simulink library "mbed_targets_stm_disco_f746"  (R2015a)
settings: Solver=ode45  StartTime=0.0  StopTime=10.0  RelTol=1e-3
libraries: mbed_targets_stm_disco_f407 x9, mbed_lib x3
settings Model: CovSFcnEnable=off  Creator=oh  LastModifiedBy=Stuv
settings DebuggingCC: SolverPrmCheckMsg=warning

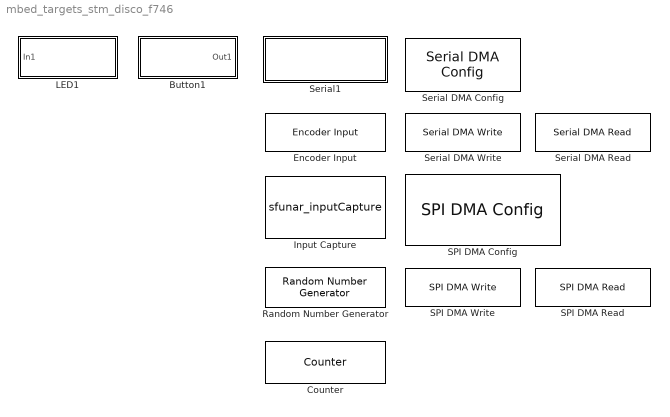
== system mbed_targets_stm_disco_f746 ==
  Button1 : Subsystem  mask{Parameter1=0}
      mask Display:
      | plot([0 0.15 0.15 0.35 0.35 0.5],[0.3 0.3 0.7 0.7 0.3 0.3])
      | port_label('output',1,['UsrBtn1']);
  Counter : mbed_targets_stm_disco_f407/Counter  TimerNumber=1  InputChannel=TI1 rising  TiPort=A  TiPin=0  TiPupd=PullNone  MaxCnt=10  Interrupt=no interrupt generation  RstEnable=off
  Encoder Input : mbed_targets_stm_disco_f407/Encoder Input  TimerNumber=TIM1  EncoderMode=TI1  Ti1Port=A  Ti1Pin=0  Ti2Port=A  Ti2Pin=0  InputMode=PullNone  Resolution=65535  SampleTime=-1
  Input Capture : S-Function  FunctionName=sfunar_inputCapture  Parameters=SampleTime, TimerNumber, Frequency, Ti1Active, Ti1Port, Ti1Pin, Ti1Pupd, Ti2Active, Ti2Port, Ti2Pin, Ti2Pupd, Ti3Active, Ti3Port, Ti3Pin, Ti3Pupd, Ti4Active, Ti4Port, Ti4Pin, Ti4Pupd, OutputMode  mask{TimerNumber=1, Frequency=1000000, OutputMode=Raw, Ti1Active=Rising, Ti1Port=A, Ti1Pin=0, Ti1Pupd=PullNone, Ti2Active=None, Ti2Port=A, Ti2Pin=0, Ti2Pupd=PullNone, Ti3Active=None, Ti3Port=A, Ti3Pin=0, Ti3Pupd=PullNone, Ti4Active=None, Ti4Port=A, Ti4Pin=0, Ti4Pupd=PullNone, SampleTime=-1}
      mask prompts: TimerNumber "Timer"; OutputMode "Output mode"; Ti1Active "Activate TI1"; Ti1Port "TI1 Port"; Ti1Pin "TI1 Pin"; Ti1Pupd "TI1 Pull type"; Ti2Active "Activate TI2"; Ti2Port "TI2 Port"; Ti2Pin "TI2 Pin"; Ti2Pupd "Ti2 Pull type"; Ti3Active "Activate TI3"; Ti3Port "TI3 Port"; Ti3Pin "TI3 Pin"; Ti3Pupd "TI3 Pull type"; Ti4Active "Activate TI4"; Ti4Port "TI4 Port"; Ti4Pin "TI4 Pin"; Ti4Pupd "TI4 Pull type"; SampleTime "Sample time (-1 for inherited):"
      mask TypeOptions TimerNumber: 1 | 2 | 3 | 4 | 5 | 8 | 9 | 10 | 11 | 12 | 13 | 14 | 15 | 16 | 17 | 20
      mask TypeOptions OutputMode: Raw | Period | Frequency | High Pulse | Low Pulse
      mask TypeOptions Ti1Active: None | Rising | Falling | Both
      mask TypeOptions Ti1Port: A | B | C | D | E | F
      mask TypeOptions Ti1Pin: 0 | 1 | 2 | 3 | 4 | 5 | 6 | 7 | 8 | 9 | 10 | 11 | 12 | 13 | 14 | 15
      mask TypeOptions Ti1Pupd: PullNone | PullUp | PullDown
      mask TypeOptions Ti2Active: None | Rising | Falling | Both
      mask TypeOptions Ti2Port: A | B | C | D | E | F
      mask TypeOptions Ti2Pin: 0 | 1 | 2 | 3 | 4 | 5 | 6 | 7 | 8 | 9 | 10 | 11 | 12 | 13 | 14 | 15
      mask TypeOptions Ti2Pupd: PullNone | PullUp | PullDown
      mask TypeOptions Ti3Active: None | Rising | Falling | Both
      mask TypeOptions Ti3Port: A | B | C | D | E | F
      mask TypeOptions Ti3Pin: 0 | 1 | 2 | 3 | 4 | 5 | 6 | 7 | 8 | 9 | 10 | 11 | 12 | 13 | 14 | 15
      mask TypeOptions Ti3Pupd: PullNone | PullUp | PullDown
      mask TypeOptions Ti4Active: None | Rising | Falling | Both
      mask TypeOptions Ti4Port: A | B | C | D | E | F
      mask TypeOptions Ti4Pin: 0 | 1 | 2 | 3 | 4 | 5 | 6 | 7 | 8 | 9 | 10 | 11 | 12 | 13 | 14 | 15
      mask TypeOptions Ti4Pupd: PullNone | PullUp | PullDown
      mask Display:
      | disp(['Timer ' num2str(TimerNumber) '\n']);
      | disp('\n Input Capture');
      | port = 1;
      | 
      | if Ti1Active > 1
      |     port_label('output',port,['P' Ti1Port+64 '.' num2str(Ti1Pin-1)]);
      |     port = port + 1;
      | end
      | 
      | if Ti2Active > 1
      |     port_label('output',port,['P' Ti2Port+64 '.' num2str(Ti2Pin-1)]);
      |     port = port + 1;
      | end
      | 
      | if Ti3Active > 1
      |     port_label('output',port,['P' Ti3Port+64 '.' num2str(Ti3Pin-1)]);
      |     port = port + 1;
      | end
      | 
      | if Ti4Active > 1
      |     port_label('output',port,['P' Ti4Port+64 '.' num2str(Ti4Pin-1)]);
      |     port = port + 1;
      | end
  LED1 : Subsystem  mask{Parameter1=0}
      mask Display:
      | plot([0.5 0.65 0.65 0.85 0.85 1],[0.3 0.3 0.7 0.7 0.3 0.3])
      | port_label('input',1,['LED1']);
  Random Number Generator : mbed_targets_stm_disco_f407/Random Number Generator  SampleTime=-1
  SPI DMA Config : mbed_targets_stm_disco_f407/SPI DMA Config  SpiPort=1  MosiPort=A  MosiPin=0  MisoPort=A  MisoPin=0  SclkPort=A  SclkPin=0  NssPort=A  NssPin=0  SlaveFlag=off  Frequency=2
  SPI DMA Read : mbed_targets_stm_disco_f407/SPI DMA Read  SpiPort=1  RxBuffer=10  PortWidth=5  SampleTime=-1
  SPI DMA Write : mbed_targets_stm_disco_f407/SPI DMA Write  SpiPort=1  numData=on  SampleTime=-1
  Serial DMA Config : mbed_targets_stm_disco_f407/Serial DMA Config  SerialPort=1  TxPort=A  TxPin=0  RxPort=A  RxPin=0  BaudRate=115200
  Serial DMA Read : mbed_targets_stm_disco_f407/Serial DMA Read  SerialPort=1  RxBuffer=10  PortWidth=5  SampleTime=-1
  Serial DMA Write : mbed_targets_stm_disco_f407/Serial DMA Write  SerialPort=1  numData=on  SampleTime=-1
  Serial1 : Subsystem  mask{Parameter1=0, BaudRate=9600}
      mask prompts: BaudRate "Baud Rate:"
      mask TypeOptions BaudRate: Serial Configuration/BaudRate
      mask Display: disp(['Serial1(USB)\nTX:PA_9, RX:PB_7'])

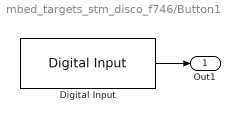
== system mbed_targets_stm_disco_f746/Button1 ==
  Digital Input : mbed_lib/GPIO/Digital Input  SParameter2=I  SParameter1=11  SParameter3=PullDefault  SampleTime=-1
  Out1 : Outport
  wires:
  Digital Input/1 -> Out1/1

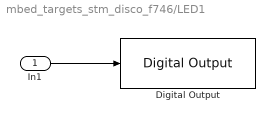
== system mbed_targets_stm_disco_f746/LED1 ==
  In1 : Inport
  Digital Output : mbed_lib/GPIO/Digital Output  SParameter2=I  SParameter1=1  SParameter3=PullDefault  SampleTime=-1
  wires:
  In1/1 -> Digital Output/1

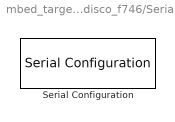
== system mbed_targets_stm_disco_f746/Serial1 ==
  Serial Configuration : mbed_lib/Serial/Serial Configuration  SerialPort=1  TXPort=A  TXPin=9  RXPort=B  RXPin=7  BaudRate=BaudRate
